simulink model "quatrosete"  (R2015a)
settings: Solver=ode45  StartTime=0.0  StopTime=1000.0  RelTol=1e-3
values from neighbouring files (symbols this model uses):
  k1 = -2    [20181030_1937.mat]
  k2 = 10    [20181030_1937.mat]
  p = 0.01    [20181030_1937.mat]
undefined symbols (not defined in the file or in its folder): kp
settings Model: Creator=Alunos  LastModifiedBy=Alunos

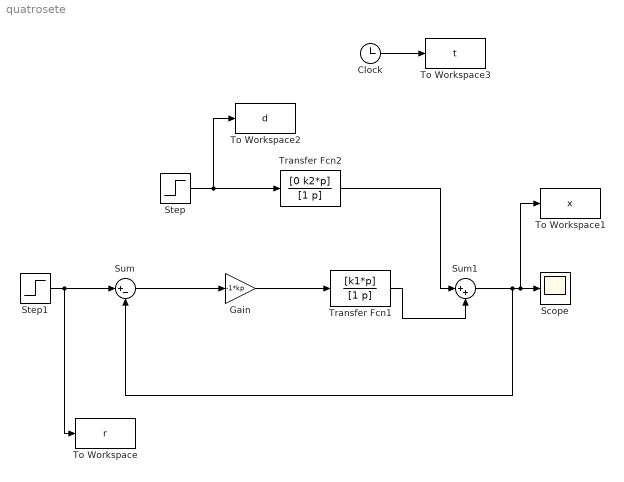
== system quatrosete ==
  Clock : Clock
  Gain : Gain  Gain=-1*kp
  Scope : Scope
  Step : Step  SampleTime=0
  Step1 : Step  After=0  SampleTime=0
  Sum : Sum  Inputs=|+-
  Sum1 : Sum  Inputs=|++
  To Workspace : ToWorkspace  VariableName=r  SampleTime=-1
  To Workspace1 : ToWorkspace  VariableName=x  SampleTime=-1
  To Workspace2 : ToWorkspace  VariableName=d  SampleTime=-1
  To Workspace3 : ToWorkspace  VariableName=t  SampleTime=-1
  Transfer Fcn1 : TransferFcn  Numerator=[k1*p]  Denominator=[1 p]
  Transfer Fcn2 : TransferFcn  Numerator=[0 k2*p]  Denominator=[1 p]
  wires:
  Gain/1 -> Transfer Fcn1/1
  Step/1 -> To Workspace2/1, Transfer Fcn2/1
  Transfer Fcn2/1 -> Sum1/1
  Transfer Fcn1/1 -> Sum1/2
  Sum/1 -> Gain/1
  Sum1/1 -> Sum/2, To Workspace1/1, Scope/1
  Clock/1 -> To Workspace3/1
  Step1/1 -> To Workspace/1, Sum/1
